simulink model "ActionPort_obs"  (Simulink 7.9)
settings: Solver=FixedStepDiscrete  SolverMode=SingleTasking  StartTime=0.0  StopTime=inf  RelTol=1e-3
PreLoadFcn:
  | if exist('tl_preloadfcn','file'), tl_preloadfcn(gcs,101); end
PostLoadFcn:
  | if exist('tl_postloadfcn','file'), tl_postloadfcn(gcs,101); end
InitFcn:
  | if exist('tlds_init','file'), tlds_init(gcs); end
StartFcn:
  | if exist('tlds_start','file'), tlds_start(gcs); end
StopFcn:
  | if exist('tlds_stop','file'), tlds_stop(gcs); end
(part 1 of 2)
PreSaveFcn:
  | if exist('tl_presavefcn','file'), tl_presavefcn(gcs); end
settings Model: TL_MAIN_DATA={'logopt',{'globalloggingmode',4},'date',736166.61526563659}  TLRevision=101  DS_PROJECTFILE=ActionPort_obs.dd  Creator=BTCJ_support  LastModifiedBy=developer  BufferReuse=off
settings OptimizationCC: BlockReduction=off  OptimizeBlockIOStorage=off  BufferReuse=off  ExpressionFolding=off  LocalBlockOutputs=off
settings DebuggingCC: StrictBusMsg=ErrorOnBusTreatedAsVector  NonBusSignalsTreatedAsBus=error
settings CodeAppCC: CustomSymbolStrType=$N$R$M_T
settings GRTTargetCC: CombineOutputUpdateFcns=off  GRTInterface=on

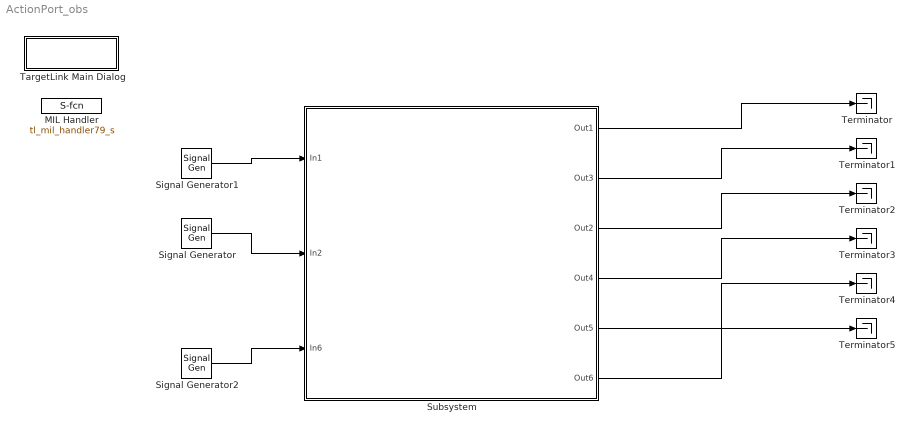
== system ActionPort_obs ==
  MIL Handler : S-Function  FunctionName=tl_mil_handler79_s  EnableBusSupport=off  mask(TL_MilHandler){data={'date',730486}}
      mask help: TargetLink MIL Handler
      mask init:
      | if get_param(0,'version') <= 8.2
      |     fname = sprintf('tl_mil_handler%d_s', 10*get_param(0,'Version'));
      | else
      | fname = sprintf('tl_mil_handler82_s');
      | end
      | set_param(gcbh,'FunctionName', fname, 'SFunctionModules','''''');
      settings: DeleteFcn=if exist('delete_tlblock','file')==2,delete_tlblock(gcbh);end  NameChangeFcn=if exist('rename_tlblock','file')==2,rename_tlblock(gcbh);end  OpenFcn=open_system(gcbh,'mask')
      mask Help: eval('if exist(''tl_online_help'',''file'') == 2, tl_online_help(''Topic'',get_param(gcbh,''MaskType'')),end')
      mask Display: disp('MIL Handler')
  Signal Generator : SignalGenerator
  Signal Generator1 : SignalGenerator
  Signal Generator2 : SignalGenerator
  Subsystem : Subsystem  Tag=TargetLink Simulation Frame
      settings: CopyFcn=if exist('tl_copyfcn','file'), tl_copyfcn(gcbh); end  NameChangeFcn=if exist('tl_framenamechangefcn','file'), tl_framenamechangefcn(gcbh); end
      settings: OpenFcn=|
      | if exist('open_tlsubsystem','file')
      |    open_tlsubsystem(gcbh);
      | else
      |    tlsubsystem = ...
      |       find_system(gcb, ...
      |       'LookUnderMasks','on', ...
      |       'FollowLinks','on', ...
      |       'Tag','MIL Subsystem');
      |    open_system(tlsubsystem);
      | end
      mask Type: TL_SimFrame
      mask Display: disp('TargetLink\nModel-\nin-the-loop\nmode')
  TargetLink Main Dialog : Subsystem  mask(TL_MainDialog){data=[]}
      mask help: TargetLink Main Dialog block: In full-featured mode it provides the main graphical user interface to TargetLink.
      mask init:
      | if exist('tl_get_blockset_mode','file')==2
      |    if strcmp(tl_get_blockset_mode,'full-featured')
      |       set_param(gcbh,'BackgroundColor','green');
      |    else
      |       set_param(gcbh,'BackgroundColor','[0.6,0.6,0.6]');
      |    end
      | else
      |    set_param(gcbh,'BackgroundColor','[0.6,0.6,0.6]');
      | end
      settings: CopyFcn=if exist('tl_copyfcn') == 2, tl_copyfcn(gcbh); end  OpenFcn=if exist('tl_open_blockdlg','file')==2,tl_open_blockdlg(gcbh);else,open_system(gcbh,'mask');end
      mask Help: eval('if exist(''tl_online_help'',''file'') == 2, tl_online_help(''Topic'',get_param(gcbh,''MaskType'')),end')
      mask Display: disp('TargetLink')
  Terminator{,1..5} (6 alike) : Terminator
  wires:
  Subsystem/1(Out1) -> Terminator/1
  Subsystem/2(Out3) -> Terminator1/1
  Subsystem/3(Out2) -> Terminator2/1
  Subsystem/4(Out4) -> Terminator3/1
  Subsystem/5(Out5) -> Terminator4/1
  Subsystem/6(Out6) -> Terminator5/1
  Signal Generator1/1 -> Subsystem/1(In1)
  Signal Generator/1 -> Subsystem/2(In2)
  Signal Generator2/1 -> Subsystem/3(In6)

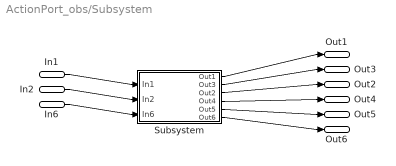
== system ActionPort_obs/Subsystem ==
  In1 : Inport
  In2 : Inport  Port=2
  In6 : Inport  Port=3
  Subsystem : Subsystem  Tag=struct('sfcnName','Subsystem_sf','subFunction','','srcSubsystem','')
      settings: OpenFcn=warndlg(get_param(gcb,'MaskHelp'),'Serious Warning');
      mask Type: TL_Enable
      mask Help: This subsystem keeps the TargetLink subsystem (subsystem with TargetLink blocks for production code generation), and is needed for the TargetLink simulation frame to work properly. DO NOT DELETE OR MODIFY IT!
  Out1 : Outport
  Out3 : Outport  Port=2
  Out2 : Outport  Port=3
  Out4 : Outport  Port=4
  Out5 : Outport  Port=5
  Out6 : Outport  Port=6
  wires:
  In1/1 -> Subsystem/1(In1)
  In2/1 -> Subsystem/2(In2)
  In6/1 -> Subsystem/3(In6)
  Subsystem/1(Out1) -> Out1/1
  Subsystem/2(Out3) -> Out3/1
  Subsystem/3(Out2) -> Out2/1
  Subsystem/4(Out4) -> Out4/1
  Subsystem/5(Out5) -> Out5/1
  Subsystem/6(Out6) -> Out6/1

== system ActionPort_obs/TargetLink Main Dialog ==
  dSPACE logo : Subsystem
      mask Display: image(ds_get_icon('dspace_logo_bg_white_l'))

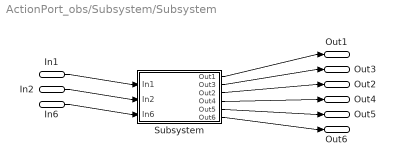
== system ActionPort_obs/Subsystem/Subsystem ==
  In1 : Inport
  In2 : Inport  Port=2
  In6 : Inport  Port=3
  Subsystem : Subsystem  Tag=MIL Subsystem  Description=a
      settings: CopyFcn=if exist('tl_copyfcn','file'), tl_copyfcn(gcbh); end  NameChangeFcn=if exist('tl_namechangefcn','file'), tl_namechangefcn(gcbh); end  DestroyFcn=if exist('update_tl_main_dlg','file'), update_tl_main_dlg('TL_subs_display'); end
      mask Type: MIL Subsystem
  Out1 : Outport
  Out3 : Outport  Port=2
  Out2 : Outport  Port=3
  Out4 : Outport  Port=4
  Out5 : Outport  Port=5
  Out6 : Outport  Port=6
  wires:
  In1/1 -> Subsystem/1(In1)
  In2/1 -> Subsystem/2(In2)
  In6/1 -> Subsystem/3(In6)
  Subsystem/1(Out1) -> Out1/1
  Subsystem/2(Out3) -> Out3/1
  Subsystem/3(Out2) -> Out2/1
  Subsystem/4(Out4) -> Out4/1
  Subsystem/5(Out5) -> Out5/1
  Subsystem/6(Out6) -> Out6/1

== system ActionPort_obs/TargetLink Main Dialog/dSPACE logo ==

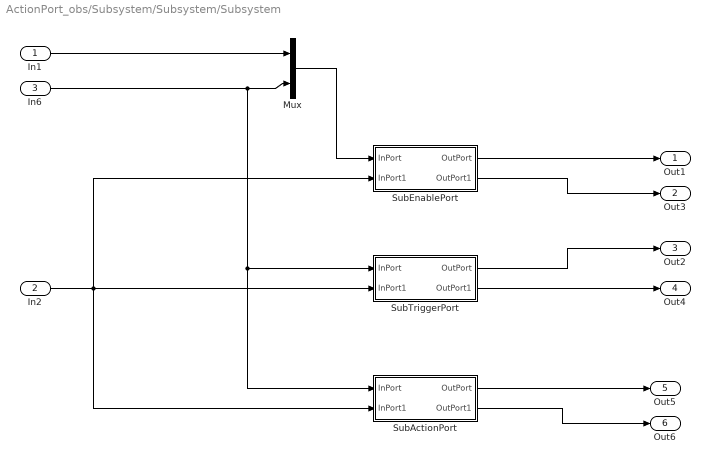
== system ActionPort_obs/Subsystem/Subsystem/Subsystem ==
  In1 : Inport  PortDimensions=1  mask(TL_Inport){data={'output',{'class','MBT_DISP'},'date',737456.38999608799}}
      settings: DeleteFcn=if exist('delete_tlblock','file')==2,delete_tlblock(gcbh);end  OpenFcn=if exist('tl_open_blockdlg','file')==2,tl_open_blockdlg(gcbh);else,open_system(gcbh,'parameter');end
      settings: CopyFcn=|
      | if exist('tl_reset_reviewflag','file')==2
      |     tl_reset_reviewflag(gcbh);
      | end
      | if exist('tl_check_ports','file')
      |     tl_check_ports(gcbh);
      | end
      settings: NameChangeFcn=|
      | if exist('rename_tlblock','file')==2,rename_tlblock(gcbh);end
      | if exist('tl_check_ports','file'), tl_check_ports(gcbh); end
      mask Help: eval(['if exist(''tl_online_help'',''file'') == 2, tl_online_help(''Topic'',''TL_Inport''),else, web([''jar:file:///'',matlabroot,''/help/toolbox/simulink/help.jar!/slref/' lower(get_param(gcbh,'Blocktype')) '.html''], ''-helpbrowser''),end'])
      mask Display: plot([0.2 0.35 NaN 0.65 0.8],[0 1 NaN 0 1]);
  In2 : Inport  Port=2  PortDimensions=1  mask(TL_Inport){data={'output',{'class','MBT_DISP'},'date',737456.38999631943}}
      settings: DeleteFcn=if exist('delete_tlblock','file')==2,delete_tlblock(gcbh);end  OpenFcn=if exist('tl_open_blockdlg','file')==2,tl_open_blockdlg(gcbh);else,open_system(gcbh,'parameter');end
      settings: CopyFcn=|
      | if exist('tl_reset_reviewflag','file')==2
      |     tl_reset_reviewflag(gcbh);
      | end
      | if exist('tl_check_ports','file')
      |     tl_check_ports(gcbh);
      | end
      settings: NameChangeFcn=|
      | if exist('rename_tlblock','file')==2,rename_tlblock(gcbh);end
      | if exist('tl_check_ports','file'), tl_check_ports(gcbh); end
      mask Help: eval(['if exist(''tl_online_help'',''file'') == 2, tl_online_help(''Topic'',''TL_Inport''),else, web([''jar:file:///'',matlabroot,''/help/toolbox/simulink/help.jar!/slref/' lower(get_param(gcbh,'Blocktype')) '.html''], ''-helpbrowser''),end'])
      mask Display: plot([0.2 0.35 NaN 0.65 0.8],[0 1 NaN 0 1]);
  In6 : Inport  Port=3  PortDimensions=1  mask(TL_Inport){data={'output',{'class','MBT_DISP'},'date',737456.38999655098}}
      settings: DeleteFcn=if exist('delete_tlblock','file')==2,delete_tlblock(gcbh);end  OpenFcn=if exist('tl_open_blockdlg','file')==2,tl_open_blockdlg(gcbh);else,open_system(gcbh,'parameter');end
      settings: CopyFcn=|
      | if exist('tl_reset_reviewflag','file')==2
      |     tl_reset_reviewflag(gcbh);
      | end
      | if exist('tl_check_ports','file')
      |     tl_check_ports(gcbh);
      | end
      settings: NameChangeFcn=|
      | if exist('rename_tlblock','file')==2,rename_tlblock(gcbh);end
      | if exist('tl_check_ports','file'), tl_check_ports(gcbh); end
      mask Help: eval(['if exist(''tl_online_help'',''file'') == 2, tl_online_help(''Topic'',''TL_Inport''),else, web([''jar:file:///'',matlabroot,''/help/toolbox/simulink/help.jar!/slref/' lower(get_param(gcbh,'Blocktype')) '.html''], ''-helpbrowser''),end'])
      mask Display: plot([0.2 0.35 NaN 0.65 0.8],[0 1 NaN 0 1]);
  Mux : Mux  Inputs=2
  SubActionPort : Subsystem
  SubEnablePort : Subsystem
  SubTriggerPort : Subsystem
  Out1 : Outport  mask(TL_Outport){data={'date',736495.67719833332}}
      settings: DeleteFcn=if exist('delete_tlblock','file')==2,delete_tlblock(gcbh);end  OpenFcn=if exist('tl_open_blockdlg','file')==2,tl_open_blockdlg(gcbh);else,open_system(gcbh,'parameter');end
      settings: CopyFcn=|
      | if exist('tl_reset_reviewflag','file')==2
      |     tl_reset_reviewflag(gcbh);
      | end
      | if exist('tl_check_ports','file')
      |     tl_check_ports(gcbh);
      | end
      settings: NameChangeFcn=|
      | if exist('rename_tlblock','file')==2,rename_tlblock(gcbh);end
      | if exist('tl_check_ports','file'), tl_check_ports(gcbh); end
      mask Help: eval(['if exist(''tl_online_help'',''file'') == 2, tl_online_help(''Topic'',''TL_Outport''),else, web([''jar:file:///'',matlabroot,''/help/toolbox/simulink/help.jar!/slref/' lower(get_param(gcbh,'Blocktype')) '.html''], ''-helpbrowser''),end'])
      mask Display: plot([0.2 0.35 NaN 0.65 0.8],[0 1 NaN 0 1]);
  Out3 : Outport  Port=2  mask(TL_Outport){data={'date',736495.6771985417}}
      settings: DeleteFcn=if exist('delete_tlblock','file')==2,delete_tlblock(gcbh);end  OpenFcn=if exist('tl_open_blockdlg','file')==2,tl_open_blockdlg(gcbh);else,open_system(gcbh,'parameter');end
      settings: CopyFcn=|
      | if exist('tl_reset_reviewflag','file')==2
      |     tl_reset_reviewflag(gcbh);
      | end
      | if exist('tl_check_ports','file')
      |     tl_check_ports(gcbh);
      | end
      settings: NameChangeFcn=|
      | if exist('rename_tlblock','file')==2,rename_tlblock(gcbh);end
      | if exist('tl_check_ports','file'), tl_check_ports(gcbh); end
      mask Help: eval(['if exist(''tl_online_help'',''file'') == 2, tl_online_help(''Topic'',''TL_Outport''),else, web([''jar:file:///'',matlabroot,''/help/toolbox/simulink/help.jar!/slref/' lower(get_param(gcbh,'Blocktype')) '.html''], ''-helpbrowser''),end'])
      mask Display: plot([0.2 0.35 NaN 0.65 0.8],[0 1 NaN 0 1]);
  Out2 : Outport  Port=3  mask(TL_Outport){data={'date',736495.67719871528}}
      settings: DeleteFcn=if exist('delete_tlblock','file')==2,delete_tlblock(gcbh);end  OpenFcn=if exist('tl_open_blockdlg','file')==2,tl_open_blockdlg(gcbh);else,open_system(gcbh,'parameter');end
      settings: CopyFcn=|
      | if exist('tl_reset_reviewflag','file')==2
      |     tl_reset_reviewflag(gcbh);
      | end
      | if exist('tl_check_ports','file')
      |     tl_check_ports(gcbh);
      | end
      settings: NameChangeFcn=|
      | if exist('rename_tlblock','file')==2,rename_tlblock(gcbh);end
      | if exist('tl_check_ports','file'), tl_check_ports(gcbh); end
      mask Help: eval(['if exist(''tl_online_help'',''file'') == 2, tl_online_help(''Topic'',''TL_Outport''),else, web([''jar:file:///'',matlabroot,''/help/toolbox/simulink/help.jar!/slref/' lower(get_param(gcbh,'Blocktype')) '.html''], ''-helpbrowser''),end'])
      mask Display: plot([0.2 0.35 NaN 0.65 0.8],[0 1 NaN 0 1]);
  Out4 : Outport  Port=4  mask(TL_Outport){data={'date',736495.67719890049}}
      settings: DeleteFcn=if exist('delete_tlblock','file')==2,delete_tlblock(gcbh);end  OpenFcn=if exist('tl_open_blockdlg','file')==2,tl_open_blockdlg(gcbh);else,open_system(gcbh,'parameter');end
      settings: CopyFcn=|
      | if exist('tl_reset_reviewflag','file')==2
      |     tl_reset_reviewflag(gcbh);
      | end
      | if exist('tl_check_ports','file')
      |     tl_check_ports(gcbh);
      | end
      settings: NameChangeFcn=|
      | if exist('rename_tlblock','file')==2,rename_tlblock(gcbh);end
      | if exist('tl_check_ports','file'), tl_check_ports(gcbh); end
      mask Help: eval(['if exist(''tl_online_help'',''file'') == 2, tl_online_help(''Topic'',''TL_Outport''),else, web([''jar:file:///'',matlabroot,''/help/toolbox/simulink/help.jar!/slref/' lower(get_param(gcbh,'Blocktype')) '.html''], ''-helpbrowser''),end'])
      mask Display: plot([0.2 0.35 NaN 0.65 0.8],[0 1 NaN 0 1]);
  Out5 : Outport  Port=5  mask(TL_Outport){data={'date',736495.67719907407}}
      settings: DeleteFcn=if exist('delete_tlblock','file')==2,delete_tlblock(gcbh);end  OpenFcn=if exist('tl_open_blockdlg','file')==2,tl_open_blockdlg(gcbh);else,open_system(gcbh,'parameter');end
      settings: CopyFcn=|
      | if exist('tl_reset_reviewflag','file')==2
      |     tl_reset_reviewflag(gcbh);
      | end
      | if exist('tl_check_ports','file')
      |     tl_check_ports(gcbh);
      | end
      settings: NameChangeFcn=|
      | if exist('rename_tlblock','file')==2,rename_tlblock(gcbh);end
      | if exist('tl_check_ports','file'), tl_check_ports(gcbh); end
      mask Help: eval(['if exist(''tl_online_help'',''file'') == 2, tl_online_help(''Topic'',''TL_Outport''),else, web([''jar:file:///'',matlabroot,''/help/toolbox/simulink/help.jar!/slref/' lower(get_param(gcbh,'Blocktype')) '.html''], ''-helpbrowser''),end'])
      mask Display: plot([0.2 0.35 NaN 0.65 0.8],[0 1 NaN 0 1]);
  Out6 : Outport  Port=6  mask(TL_Outport){data={'date',736495.67719924764}}
      settings: DeleteFcn=if exist('delete_tlblock','file')==2,delete_tlblock(gcbh);end  OpenFcn=if exist('tl_open_blockdlg','file')==2,tl_open_blockdlg(gcbh);else,open_system(gcbh,'parameter');end
      settings: CopyFcn=|
      | if exist('tl_reset_reviewflag','file')==2
      |     tl_reset_reviewflag(gcbh);
      | end
      | if exist('tl_check_ports','file')
      |     tl_check_ports(gcbh);
      | end
      settings: NameChangeFcn=|
      | if exist('rename_tlblock','file')==2,rename_tlblock(gcbh);end
      | if exist('tl_check_ports','file'), tl_check_ports(gcbh); end
      mask Help: eval(['if exist(''tl_online_help'',''file'') == 2, tl_online_help(''Topic'',''TL_Outport''),else, web([''jar:file:///'',matlabroot,''/help/toolbox/simulink/help.jar!/slref/' lower(get_param(gcbh,'Blocktype')) '.html''], ''-helpbrowser''),end'])
      mask Display: plot([0.2 0.35 NaN 0.65 0.8],[0 1 NaN 0 1]);
  wires:
  In6/1 -> SubActionPort/1(InPort), SubTriggerPort/1(InPort), Mux/2
  In1/1 -> Mux/1
  Mux/1 -> SubEnablePort/1(InPort)
  In2/1 -> SubActionPort/2(InPort1), SubTriggerPort/2(InPort1), SubEnablePort/2(InPort1)
  SubEnablePort/1(OutPort) -> Out1/1
  SubEnablePort/2(OutPort1) -> Out3/1
  SubTriggerPort/1(OutPort) -> Out2/1
  SubTriggerPort/2(OutPort1) -> Out4/1
  SubActionPort/1(OutPort) -> Out5/1
  SubActionPort/2(OutPort1) -> Out6/1

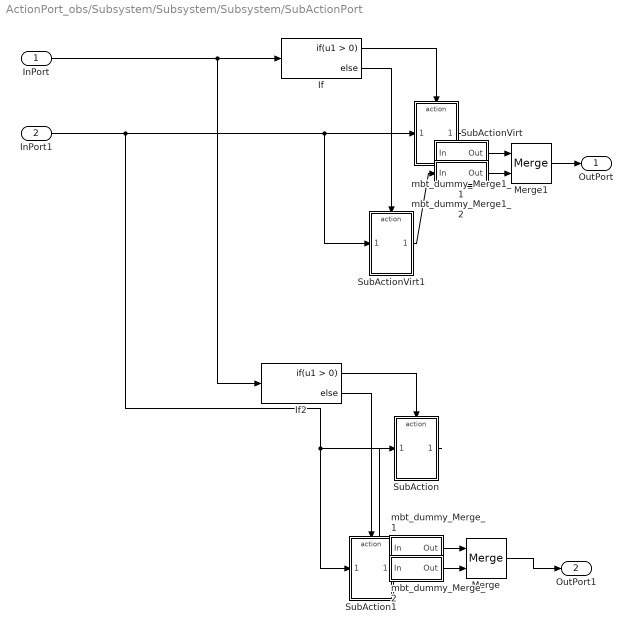
== system ActionPort_obs/Subsystem/Subsystem/Subsystem/SubActionPort ==
  InPort : Inport
      settings: CopyFcn=if exist('tl_reset_reviewflag') == 2, tl_reset_reviewflag(gcbh); end  DeleteFcn=if exist('delete_tlblock','file')==2,delete_tlblock(gcbh);end  NameChangeFcn=if exist('rename_tlblock','file')==2,rename_tlblock(gcbh);end  OpenFcn=if exist('tl_open_blockdlg','file')==2,tl_open_blockdlg(gcbh);else,open_system(gcbh,'parameter');end
  InPort1 : Inport  Port=2
      settings: CopyFcn=if exist('tl_reset_reviewflag') == 2, tl_reset_reviewflag(gcbh); end  DeleteFcn=if exist('delete_tlblock','file')==2,delete_tlblock(gcbh);end  NameChangeFcn=if exist('rename_tlblock','file')==2,rename_tlblock(gcbh);end  OpenFcn=if exist('tl_open_blockdlg','file')==2,tl_open_blockdlg(gcbh);else,open_system(gcbh,'parameter');end
  If : If
  If2 : If
  Merge : Merge  InitialOutput=[0]  mask(TL_Merge){data={'date',736495.67979597219}}
      settings: CopyFcn=if exist('tl_reset_reviewflag','file')==2,tl_reset_reviewflag(gcbh);end  DeleteFcn=if exist('delete_tlblock','file')==2,delete_tlblock(gcbh);end  NameChangeFcn=if exist('rename_tlblock','file')==2,rename_tlblock(gcbh);end  OpenFcn=if exist('tl_open_blockdlg','file')==2,tl_open_blockdlg(gcbh);else,open_system(gcbh,'parameter');end
      mask Help: eval(['if exist(''tl_online_help'',''file'') == 2, tl_online_help(''Topic'',''TL_Merge''),else, web([''jar:file:///'',matlabroot,''/help/toolbox/simulink/help.jar!/slref/' lower(get_param(gcbh,'Blocktype')) '.html''], ''-helpbrowser''),end'])
      mask Display: plot([-0.05, 1.05, NaN, -0.05, 1.05],[.01, .01, NaN, .99, .99])
  Merge1 : Merge  InitialOutput=[0]  mask(TL_Merge){data={'date',736495.679845787}}
      settings: CopyFcn=if exist('tl_reset_reviewflag','file')==2,tl_reset_reviewflag(gcbh);end  DeleteFcn=if exist('delete_tlblock','file')==2,delete_tlblock(gcbh);end  NameChangeFcn=if exist('rename_tlblock','file')==2,rename_tlblock(gcbh);end  OpenFcn=if exist('tl_open_blockdlg','file')==2,tl_open_blockdlg(gcbh);else,open_system(gcbh,'parameter');end
      mask Help: eval(['if exist(''tl_online_help'',''file'') == 2, tl_online_help(''Topic'',''TL_Merge''),else, web([''jar:file:///'',matlabroot,''/help/toolbox/simulink/help.jar!/slref/' lower(get_param(gcbh,'Blocktype')) '.html''], ''-helpbrowser''),end'])
      mask Display: plot([-0.05, 1.05, NaN, -0.05, 1.05],[.01, .01, NaN, .99, .99])
  SubAction : Subsystem
  SubAction1 : Subsystem
  SubActionVirt : Subsystem
  SubActionVirt1 : Subsystem
  mbt_dummy_Merge1_1 : Subsystem  Tag=et_enhanced_observability
      mask Type: MBT_DUMMY_BLOCK
      mask Display: text(0.1, 0.5, 'MBT_DUMMY')
  mbt_dummy_Merge1_2 : Subsystem  Tag=et_enhanced_observability
      mask Type: MBT_DUMMY_BLOCK
      mask Display: text(0.1, 0.5, 'MBT_DUMMY')
  mbt_dummy_Merge_1 : Subsystem  Tag=et_enhanced_observability
      mask Type: MBT_DUMMY_BLOCK
      mask Display: text(0.1, 0.5, 'MBT_DUMMY')
  mbt_dummy_Merge_2 : Subsystem  Tag=et_enhanced_observability
      mask Type: MBT_DUMMY_BLOCK
      mask Display: text(0.1, 0.5, 'MBT_DUMMY')
  OutPort : Outport
      settings: CopyFcn=if exist('tl_reset_reviewflag') == 2, tl_reset_reviewflag(gcbh); end  DeleteFcn=if exist('delete_tlblock','file')==2,delete_tlblock(gcbh);end  NameChangeFcn=if exist('rename_tlblock','file')==2,rename_tlblock(gcbh);end  OpenFcn=if exist('tl_open_blockdlg','file')==2,tl_open_blockdlg(gcbh);else,open_system(gcbh,'parameter');end
  OutPort1 : Outport  Port=2
      settings: CopyFcn=if exist('tl_reset_reviewflag') == 2, tl_reset_reviewflag(gcbh); end  DeleteFcn=if exist('delete_tlblock','file')==2,delete_tlblock(gcbh);end  NameChangeFcn=if exist('rename_tlblock','file')==2,rename_tlblock(gcbh);end  OpenFcn=if exist('tl_open_blockdlg','file')==2,tl_open_blockdlg(gcbh);else,open_system(gcbh,'parameter');end
  wires:
  InPort1/1 -> SubAction1/1(In1), SubAction/1(In1), SubActionVirt1/1(In1), SubActionVirt/1(In1)
  If2/1 -> SubAction/Action
  If/1 -> SubActionVirt/Action
  InPort/1 -> If2/1, If/1
  If2/2 -> SubAction1/Action
  Merge/1 -> OutPort1/1
  If/2 -> SubActionVirt1/Action
  Merge1/1 -> OutPort/1
  SubAction/1(Out1) -> mbt_dummy_Merge_1/1(In)
  mbt_dummy_Merge_1/1(Out) -> Merge/1
  SubAction1/1(Out1) -> mbt_dummy_Merge_2/1(In)
  mbt_dummy_Merge_2/1(Out) -> Merge/2
  SubActionVirt/1(Out1) -> mbt_dummy_Merge1_1/1(In)
  mbt_dummy_Merge1_1/1(Out) -> Merge1/1
  SubActionVirt1/1(Out1) -> mbt_dummy_Merge1_2/1(In)
  mbt_dummy_Merge1_2/1(Out) -> Merge1/2

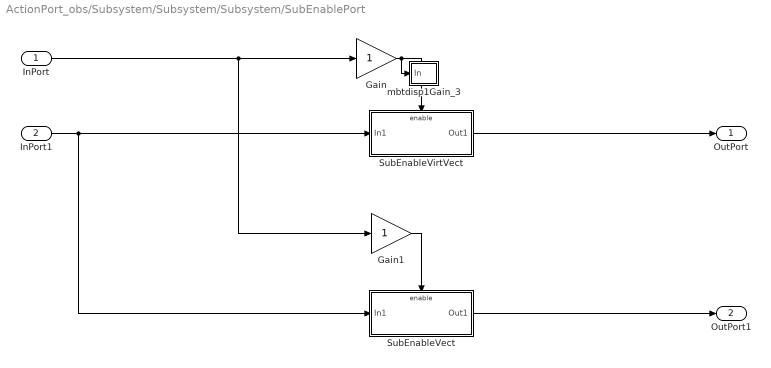
== system ActionPort_obs/Subsystem/Subsystem/Subsystem/SubEnablePort ==
  InPort : Inport
      settings: CopyFcn=if exist('tl_reset_reviewflag') == 2, tl_reset_reviewflag(gcbh); end  DeleteFcn=if exist('delete_tlblock','file')==2,delete_tlblock(gcbh);end  NameChangeFcn=if exist('rename_tlblock','file')==2,rename_tlblock(gcbh);end  OpenFcn=if exist('tl_open_blockdlg','file')==2,tl_open_blockdlg(gcbh);else,open_system(gcbh,'parameter');end
  InPort1 : Inport  Port=2
      settings: CopyFcn=if exist('tl_reset_reviewflag') == 2, tl_reset_reviewflag(gcbh); end  DeleteFcn=if exist('delete_tlblock','file')==2,delete_tlblock(gcbh);end  NameChangeFcn=if exist('rename_tlblock','file')==2,rename_tlblock(gcbh);end  OpenFcn=if exist('tl_open_blockdlg','file')==2,tl_open_blockdlg(gcbh);else,open_system(gcbh,'parameter');end
  Gain : Gain  mask(TL_Gain){data={'date',736495.67750707176}}
      settings: CopyFcn=if exist('tl_reset_reviewflag','file')==2,tl_reset_reviewflag(gcbh);end  DeleteFcn=if exist('delete_tlblock','file')==2,delete_tlblock(gcbh);end  NameChangeFcn=if exist('rename_tlblock','file')==2,rename_tlblock(gcbh);end  OpenFcn=if exist('tl_open_blockdlg','file')==2,tl_open_blockdlg(gcbh);else,open_system(gcbh,'parameter');end
      mask Help: eval(['if exist(''tl_online_help'',''file'') == 2, tl_online_help(''Topic'',''TL_Gain''),else, web([''jar:file:///'',matlabroot,''/help/toolbox/simulink/help.jar!/slref/' lower(get_param(gcbh,'Blocktype')) '.html''], ''-helpbrowser''),end'])
      mask Display: plot([0, .9, 0],[.05, .5, .95])
  Gain1 : Gain  mask(TL_Gain){data={'date',736495.67750723381}}
      settings: CopyFcn=if exist('tl_reset_reviewflag','file')==2,tl_reset_reviewflag(gcbh);end  DeleteFcn=if exist('delete_tlblock','file')==2,delete_tlblock(gcbh);end  NameChangeFcn=if exist('rename_tlblock','file')==2,rename_tlblock(gcbh);end  OpenFcn=if exist('tl_open_blockdlg','file')==2,tl_open_blockdlg(gcbh);else,open_system(gcbh,'parameter');end
      mask Help: eval(['if exist(''tl_online_help'',''file'') == 2, tl_online_help(''Topic'',''TL_Gain''),else, web([''jar:file:///'',matlabroot,''/help/toolbox/simulink/help.jar!/slref/' lower(get_param(gcbh,'Blocktype')) '.html''], ''-helpbrowser''),end'])
      mask Display: plot([0, .9, 0],[.05, .5, .95])
  SubEnableVect : Subsystem
  SubEnableVirtVect : Subsystem
  mbtdisp1Gain_3 : Subsystem  Tag=et_enhanced_observability
      mask Type: MBT_DISP_BLOCK
      mask Display: text(0.1, 0.5, 'MBT_DISP')
  OutPort : Outport
      settings: CopyFcn=if exist('tl_reset_reviewflag') == 2, tl_reset_reviewflag(gcbh); end  DeleteFcn=if exist('delete_tlblock','file')==2,delete_tlblock(gcbh);end  NameChangeFcn=if exist('rename_tlblock','file')==2,rename_tlblock(gcbh);end  OpenFcn=if exist('tl_open_blockdlg','file')==2,tl_open_blockdlg(gcbh);else,open_system(gcbh,'parameter');end
  OutPort1 : Outport  Port=2
      settings: CopyFcn=if exist('tl_reset_reviewflag') == 2, tl_reset_reviewflag(gcbh); end  DeleteFcn=if exist('delete_tlblock','file')==2,delete_tlblock(gcbh);end  NameChangeFcn=if exist('rename_tlblock','file')==2,rename_tlblock(gcbh);end  OpenFcn=if exist('tl_open_blockdlg','file')==2,tl_open_blockdlg(gcbh);else,open_system(gcbh,'parameter');end
  wires:
  InPort1/1 -> SubEnableVect/1(In1), SubEnableVirtVect/1(In1)
  InPort/1 -> Gain1/1, Gain/1
  SubEnableVirtVect/1(Out1) -> OutPort/1
  SubEnableVect/1(Out1) -> OutPort1/1
  Gain/1 -> SubEnableVirtVect/Enable, mbtdisp1Gain_3/1(In)
  Gain1/1 -> SubEnableVect/Enable

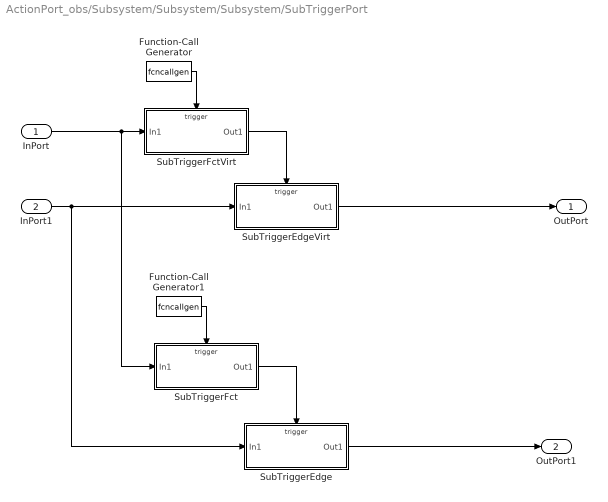
== system ActionPort_obs/Subsystem/Subsystem/Subsystem/SubTriggerPort ==
  InPort : Inport
      settings: CopyFcn=if exist('tl_reset_reviewflag') == 2, tl_reset_reviewflag(gcbh); end  DeleteFcn=if exist('delete_tlblock','file')==2,delete_tlblock(gcbh);end  NameChangeFcn=if exist('rename_tlblock','file')==2,rename_tlblock(gcbh);end  OpenFcn=if exist('tl_open_blockdlg','file')==2,tl_open_blockdlg(gcbh);else,open_system(gcbh,'parameter');end
  InPort1 : Inport  Port=2
      settings: CopyFcn=if exist('tl_reset_reviewflag') == 2, tl_reset_reviewflag(gcbh); end  DeleteFcn=if exist('delete_tlblock','file')==2,delete_tlblock(gcbh);end  NameChangeFcn=if exist('rename_tlblock','file')==2,rename_tlblock(gcbh);end  OpenFcn=if exist('tl_open_blockdlg','file')==2,tl_open_blockdlg(gcbh);else,open_system(gcbh,'parameter');end
  Function-Call Generator : S-Function  FunctionName=fcncallgen  Parameters=sample_time,numberOfIterations  EnableBusSupport=off  mask(Function-Call Generator){sample_time=2, numberOfIterations=1}
      mask prompts: sample_time "Simulink:masks:SampleTime_MP"; numberOfIterations "Simulink:masks:NumberOfIterations_MP"
      mask help: Simulink:masks:FunctionCallGenerator_MD
      mask init:
      | if ~isempty(numberOfIterations) & length(numberOfIterations) == 1 & (numberOfIterations > 1),
      | str=sprintf('iterate I = 1:%d',numberOfIterations);
      | else, str = 'f()';
      | end;
      mask Help: This block executes a function-call subsystem at the rate specified by the sample time and a specified number of times.
      mask Display: disp(str)
  Function-Call Generator1 : S-Function  FunctionName=fcncallgen  Parameters=sample_time,numberOfIterations  EnableBusSupport=off  mask(Function-Call Generator){sample_time=2, numberOfIterations=1}
      mask prompts: sample_time "Simulink:masks:SampleTime_MP"; numberOfIterations "Simulink:masks:NumberOfIterations_MP"
      mask help: Simulink:masks:FunctionCallGenerator_MD
      mask init:
      | if ~isempty(numberOfIterations) & length(numberOfIterations) == 1 & (numberOfIterations > 1),
      | str=sprintf('iterate I = 1:%d',numberOfIterations);
      | else, str = 'f()';
      | end;
      mask Help: This block executes a function-call subsystem at the rate specified by the sample time and a specified number of times.
      mask Display: disp(str)
  SubTriggerEdge : Subsystem
  SubTriggerEdgeVirt : Subsystem
  SubTriggerFct : Subsystem
  SubTriggerFctVirt : Subsystem
  OutPort : Outport
      settings: CopyFcn=if exist('tl_reset_reviewflag') == 2, tl_reset_reviewflag(gcbh); end  DeleteFcn=if exist('delete_tlblock','file')==2,delete_tlblock(gcbh);end  NameChangeFcn=if exist('rename_tlblock','file')==2,rename_tlblock(gcbh);end  OpenFcn=if exist('tl_open_blockdlg','file')==2,tl_open_blockdlg(gcbh);else,open_system(gcbh,'parameter');end
  OutPort1 : Outport  Port=2
      settings: CopyFcn=if exist('tl_reset_reviewflag') == 2, tl_reset_reviewflag(gcbh); end  DeleteFcn=if exist('delete_tlblock','file')==2,delete_tlblock(gcbh);end  NameChangeFcn=if exist('rename_tlblock','file')==2,rename_tlblock(gcbh);end  OpenFcn=if exist('tl_open_blockdlg','file')==2,tl_open_blockdlg(gcbh);else,open_system(gcbh,'parameter');end
  wires:
  InPort/1 -> SubTriggerFct/1(In1), SubTriggerFctVirt/1(In1)
  SubTriggerFctVirt/1(Out1) -> SubTriggerEdgeVirt/Trigger
  Function-Call Generator/1 -> SubTriggerFctVirt/Trigger
  SubTriggerEdgeVirt/1(Out1) -> OutPort/1
  SubTriggerFct/1(Out1) -> SubTriggerEdge/Trigger
  Function-Call Generator1/1 -> SubTriggerFct/Trigger
  SubTriggerEdge/1(Out1) -> OutPort1/1
  InPort1/1 -> SubTriggerEdge/1(In1), SubTriggerEdgeVirt/1(In1)

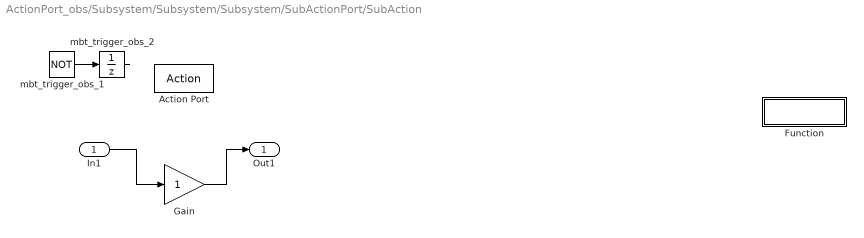
== system ActionPort_obs/Subsystem/Subsystem/Subsystem/SubActionPort/SubAction ==
  In1 : Inport
  Action Port : ActionPort  ActionType=then
  Function : Subsystem  LoadFcn=if exist('tl_loadfcn','file')==2,tl_loadfcn(gcbh);end  mask(TL_Function){data={'date',730486}}
      mask help: TargetLink Function block: It is used to generate code for a subsystem in a separate C function. In full-featured mode it provides an graphical user interface.
      mask init:
      | hBlock = gcbh;
      | if exist('tl_get_blockset_mode','file')==2
      |    if strcmp(tl_get_blockset_mode,'full-featured')
      |       set_param(hBlock,'BackgroundColor','green');
      |    else
      |       set_param(hBlock,'BackgroundColor','[0.6,0.6,0.6]');
      |    end
      | else
      |    set_param(hBlock,'BackgroundColor','[0.6,0.6,0.6]');
      | end
      |  
      | if exist('tl_add_swcparameter','file')==2
      |     tl_add_swcparameter(hBlock);
      | end
      settings: DeleteFcn=if exist('delete_tlblock','file')==2,delete_tlblock(gcbh);end  NameChangeFcn=if exist('rename_tlblock','file')==2,rename_tlblock(gcbh);end  OpenFcn=if exist('tl_open_blockdlg','file')==2,tl_open_blockdlg(gcbh);else,open_system(gcbh,'mask');end
      mask Help: eval('if exist(''tl_online_help'',''file'') == 2, tl_online_help(''Topic'',get_param(gcbh,''MaskType'')),end')
      mask Display: disp('FUNCTION')
  Gain : Gain  mask(TL_Gain){data={'date',736495.67856915505}}
      settings: CopyFcn=if exist('tl_reset_reviewflag','file')==2,tl_reset_reviewflag(gcbh);end  DeleteFcn=if exist('delete_tlblock','file')==2,delete_tlblock(gcbh);end  NameChangeFcn=if exist('rename_tlblock','file')==2,rename_tlblock(gcbh);end  OpenFcn=if exist('tl_open_blockdlg','file')==2,tl_open_blockdlg(gcbh);else,open_system(gcbh,'parameter');end
      mask Help: eval(['if exist(''tl_online_help'',''file'') == 2, tl_online_help(''Topic'',''TL_Gain''),else, web([''jar:file:///'',matlabroot,''/help/toolbox/simulink/help.jar!/slref/' lower(get_param(gcbh,'Blocktype')) '.html''], ''-helpbrowser''),end'])
      mask Display: plot([0, .9, 0],[.05, .5, .95])
  mbt_trigger_obs_1 : Logic  Tag=mbt_add_trigger_obs  Operator=NOT  Inputs=1  AllPortsSameDT=off  OutDataTypeStr=boolean  mask(TL_LogicalOperator){data={'output',{'class','MBT_DISP'},'date',737456.38998781249}}
      settings: DeleteFcn=if exist('delete_tlblock','file')==2,delete_tlblock(gcbh);end  NameChangeFcn=if exist('rename_tlblock','file')==2,rename_tlblock(gcbh);end  OpenFcn=if exist('tl_open_blockdlg','file')==2,tl_open_blockdlg(gcbh);else,open_system(gcbh,'parameter');end
      mask Help: eval(['if exist(''tl_online_help'',''file'') == 2, tl_online_help(''Topic'',''TL_LogicalOperator''),else, web([''jar:file:///'',matlabroot,''/help/toolbox/simulink/help.jar!/slref/' lower(get_param(gcbh,'Blocktype')) '.html''], ''-helpbrowser''),end'])
      mask Display: plot([-0.05, 1.05, NaN, -0.05, 1.05],[.01, .01, NaN, .99, .99])
  mbt_trigger_obs_2 : UnitDelay  Tag=mbt_add_trigger_obs  SampleTime=-1  mask(TL_UnitDelay){data={'output',{'type','Bool'},'state',{'type','Bool'},'date',737456.38998839119}}
      settings: CopyFcn=if exist('tl_reset_reviewflag') == 2, tl_reset_reviewflag(gcbh); end  DeleteFcn=if exist('delete_tlblock','file')==2,delete_tlblock(gcbh);end  NameChangeFcn=if exist('rename_tlblock','file')==2,rename_tlblock(gcbh);end  OpenFcn=if exist('tl_open_blockdlg','file')==2,tl_open_blockdlg(gcbh);else,open_system(gcbh,'parameter');end
      mask Help: eval(['if exist(''tl_online_help'',''file'') == 2, tl_online_help(''Topic'',''TL_UnitDelay''),else, web([''jar:file:///'',matlabroot,''/help/toolbox/simulink/help.jar!/slref/' lower(get_param(gcbh,'Blocktype')) '.html''], ''-helpbrowser''),end'])
      mask Display: plot([-0.05, 1.05, NaN, -0.05, 1.05],[.01, .01, NaN, .99, .99])
  Out1 : Outport  InitialOutput=0
  wires:
  In1/1 -> Gain/1
  Gain/1 -> Out1/1
  mbt_trigger_obs_1/1 -> mbt_trigger_obs_2/1
  mbt_trigger_obs_2/1 -> mbt_trigger_obs_1/1

== system ActionPort_obs/Subsystem/Subsystem/Subsystem/SubActionPort/SubAction1 ==
  In1 : Inport
  Action Port : ActionPort  ActionType=else
  Function : Subsystem  LoadFcn=if exist('tl_loadfcn','file')==2,tl_loadfcn(gcbh);end  mask(TL_Function){data={'date',730486}}
      mask help: TargetLink Function block: It is used to generate code for a subsystem in a separate C function. In full-featured mode it provides an graphical user interface.
      mask init: same as ActionPort_obs/Subsystem/Subsystem/Subsystem/SubActionPort/SubAction/Function
      settings: DeleteFcn=if exist('delete_tlblock','file')==2,delete_tlblock(gcbh);end  NameChangeFcn=if exist('rename_tlblock','file')==2,rename_tlblock(gcbh);end  OpenFcn=if exist('tl_open_blockdlg','file')==2,tl_open_blockdlg(gcbh);else,open_system(gcbh,'mask');end
      mask Help: eval('if exist(''tl_online_help'',''file'') == 2, tl_online_help(''Topic'',get_param(gcbh,''MaskType'')),end')
      mask Display: disp('FUNCTION')
  Gain : Gain  mask(TL_Gain){data={'date',736495.678753588}}
      settings: CopyFcn=if exist('tl_reset_reviewflag','file')==2,tl_reset_reviewflag(gcbh);end  DeleteFcn=if exist('delete_tlblock','file')==2,delete_tlblock(gcbh);end  NameChangeFcn=if exist('rename_tlblock','file')==2,rename_tlblock(gcbh);end  OpenFcn=if exist('tl_open_blockdlg','file')==2,tl_open_blockdlg(gcbh);else,open_system(gcbh,'parameter');end
      mask Help: eval(['if exist(''tl_online_help'',''file'') == 2, tl_online_help(''Topic'',''TL_Gain''),else, web([''jar:file:///'',matlabroot,''/help/toolbox/simulink/help.jar!/slref/' lower(get_param(gcbh,'Blocktype')) '.html''], ''-helpbrowser''),end'])
      mask Display: plot([0, .9, 0],[.05, .5, .95])
  mbt_trigger_obs_1 : Logic  Tag=mbt_add_trigger_obs  Operator=NOT  Inputs=1  AllPortsSameDT=off  OutDataTypeStr=boolean  mask(TL_LogicalOperator){data={'output',{'class','MBT_DISP'},'date',737456.38999358797}}
      settings: DeleteFcn=if exist('delete_tlblock','file')==2,delete_tlblock(gcbh);end  NameChangeFcn=if exist('rename_tlblock','file')==2,rename_tlblock(gcbh);end  OpenFcn=if exist('tl_open_blockdlg','file')==2,tl_open_blockdlg(gcbh);else,open_system(gcbh,'parameter');end
      mask Help: eval(['if exist(''tl_online_help'',''file'') == 2, tl_online_help(''Topic'',''TL_LogicalOperator''),else, web([''jar:file:///'',matlabroot,''/help/toolbox/simulink/help.jar!/slref/' lower(get_param(gcbh,'Blocktype')) '.html''], ''-helpbrowser''),end'])
      mask Display: plot([-0.05, 1.05, NaN, -0.05, 1.05],[.01, .01, NaN, .99, .99])
  mbt_trigger_obs_2 : UnitDelay  Tag=mbt_add_trigger_obs  SampleTime=-1  mask(TL_UnitDelay){data={'output',{'type','Bool'},'state',{'type','Bool'},'date',737456.38999415515}}
      settings: CopyFcn=if exist('tl_reset_reviewflag') == 2, tl_reset_reviewflag(gcbh); end  DeleteFcn=if exist('delete_tlblock','file')==2,delete_tlblock(gcbh);end  NameChangeFcn=if exist('rename_tlblock','file')==2,rename_tlblock(gcbh);end  OpenFcn=if exist('tl_open_blockdlg','file')==2,tl_open_blockdlg(gcbh);else,open_system(gcbh,'parameter');end
      mask Help: eval(['if exist(''tl_online_help'',''file'') == 2, tl_online_help(''Topic'',''TL_UnitDelay''),else, web([''jar:file:///'',matlabroot,''/help/toolbox/simulink/help.jar!/slref/' lower(get_param(gcbh,'Blocktype')) '.html''], ''-helpbrowser''),end'])
      mask Display: plot([-0.05, 1.05, NaN, -0.05, 1.05],[.01, .01, NaN, .99, .99])
  Out1 : Outport  InitialOutput=0
  wires:
  In1/1 -> Gain/1
  Gain/1 -> Out1/1
  mbt_trigger_obs_1/1 -> mbt_trigger_obs_2/1
  mbt_trigger_obs_2/1 -> mbt_trigger_obs_1/1

== system ActionPort_obs/Subsystem/Subsystem/Subsystem/SubActionPort/SubActionVirt ==
  In1 : Inport
  Action Port : ActionPort  ActionType=then
  Gain : Gain  mask(TL_Gain){data={'date',736495.67814083328}}
      settings: CopyFcn=if exist('tl_reset_reviewflag','file')==2,tl_reset_reviewflag(gcbh);end  DeleteFcn=if exist('delete_tlblock','file')==2,delete_tlblock(gcbh);end  NameChangeFcn=if exist('rename_tlblock','file')==2,rename_tlblock(gcbh);end  OpenFcn=if exist('tl_open_blockdlg','file')==2,tl_open_blockdlg(gcbh);else,open_system(gcbh,'parameter');end
      mask Help: eval(['if exist(''tl_online_help'',''file'') == 2, tl_online_help(''Topic'',''TL_Gain''),else, web([''jar:file:///'',matlabroot,''/help/toolbox/simulink/help.jar!/slref/' lower(get_param(gcbh,'Blocktype')) '.html''], ''-helpbrowser''),end'])
      mask Display: plot([0, .9, 0],[.05, .5, .95])
  mbt_trigger_obs_1 : Logic  Tag=mbt_add_trigger_obs  Operator=NOT  Inputs=1  AllPortsSameDT=off  OutDataTypeStr=boolean  mask(TL_LogicalOperator){data={'output',{'class','MBT_DISP'},'date',737456.38998442132}}
      settings: DeleteFcn=if exist('delete_tlblock','file')==2,delete_tlblock(gcbh);end  NameChangeFcn=if exist('rename_tlblock','file')==2,rename_tlblock(gcbh);end  OpenFcn=if exist('tl_open_blockdlg','file')==2,tl_open_blockdlg(gcbh);else,open_system(gcbh,'parameter');end
      mask Help: eval(['if exist(''tl_online_help'',''file'') == 2, tl_online_help(''Topic'',''TL_LogicalOperator''),else, web([''jar:file:///'',matlabroot,''/help/toolbox/simulink/help.jar!/slref/' lower(get_param(gcbh,'Blocktype')) '.html''], ''-helpbrowser''),end'])
      mask Display: plot([-0.05, 1.05, NaN, -0.05, 1.05],[.01, .01, NaN, .99, .99])
  mbt_trigger_obs_2 : UnitDelay  Tag=mbt_add_trigger_obs  SampleTime=-1  mask(TL_UnitDelay){data={'output',{'type','Bool'},'state',{'type','Bool'},'date',737456.38998500002}}
      settings: CopyFcn=if exist('tl_reset_reviewflag') == 2, tl_reset_reviewflag(gcbh); end  DeleteFcn=if exist('delete_tlblock','file')==2,delete_tlblock(gcbh);end  NameChangeFcn=if exist('rename_tlblock','file')==2,rename_tlblock(gcbh);end  OpenFcn=if exist('tl_open_blockdlg','file')==2,tl_open_blockdlg(gcbh);else,open_system(gcbh,'parameter');end
      mask Help: eval(['if exist(''tl_online_help'',''file'') == 2, tl_online_help(''Topic'',''TL_UnitDelay''),else, web([''jar:file:///'',matlabroot,''/help/toolbox/simulink/help.jar!/slref/' lower(get_param(gcbh,'Blocktype')) '.html''], ''-helpbrowser''),end'])
      mask Display: plot([-0.05, 1.05, NaN, -0.05, 1.05],[.01, .01, NaN, .99, .99])
  Out1 : Outport  InitialOutput=0
  wires:
  In1/1 -> Gain/1
  Gain/1 -> Out1/1
  mbt_trigger_obs_1/1 -> mbt_trigger_obs_2/1
  mbt_trigger_obs_2/1 -> mbt_trigger_obs_1/1

== system ActionPort_obs/Subsystem/Subsystem/Subsystem/SubActionPort/SubActionVirt1 ==
  In1 : Inport
  Action Port : ActionPort  ActionType=else
  Gain : Gain  mask(TL_Gain){data={'date',736495.67832232639}}
      settings: CopyFcn=if exist('tl_reset_reviewflag','file')==2,tl_reset_reviewflag(gcbh);end  DeleteFcn=if exist('delete_tlblock','file')==2,delete_tlblock(gcbh);end  NameChangeFcn=if exist('rename_tlblock','file')==2,rename_tlblock(gcbh);end  OpenFcn=if exist('tl_open_blockdlg','file')==2,tl_open_blockdlg(gcbh);else,open_system(gcbh,'parameter');end
      mask Help: eval(['if exist(''tl_online_help'',''file'') == 2, tl_online_help(''Topic'',''TL_Gain''),else, web([''jar:file:///'',matlabroot,''/help/toolbox/simulink/help.jar!/slref/' lower(get_param(gcbh,'Blocktype')) '.html''], ''-helpbrowser''),end'])
      mask Display: plot([0, .9, 0],[.05, .5, .95])
  mbt_trigger_obs_1 : Logic  Tag=mbt_add_trigger_obs  Operator=NOT  Inputs=1  AllPortsSameDT=off  OutDataTypeStr=boolean  mask(TL_LogicalOperator){data={'output',{'class','MBT_DISP'},'date',737456.38999011577}}
      settings: DeleteFcn=if exist('delete_tlblock','file')==2,delete_tlblock(gcbh);end  NameChangeFcn=if exist('rename_tlblock','file')==2,rename_tlblock(gcbh);end  OpenFcn=if exist('tl_open_blockdlg','file')==2,tl_open_blockdlg(gcbh);else,open_system(gcbh,'parameter');end
      mask Help: eval(['if exist(''tl_online_help'',''file'') == 2, tl_online_help(''Topic'',''TL_LogicalOperator''),else, web([''jar:file:///'',matlabroot,''/help/toolbox/simulink/help.jar!/slref/' lower(get_param(gcbh,'Blocktype')) '.html''], ''-helpbrowser''),end'])
      mask Display: plot([-0.05, 1.05, NaN, -0.05, 1.05],[.01, .01, NaN, .99, .99])
  mbt_trigger_obs_2 : UnitDelay  Tag=mbt_add_trigger_obs  SampleTime=-1  mask(TL_UnitDelay){data={'output',{'type','Bool'},'state',{'type','Bool'},'date',737456.38999069447}}
      settings: CopyFcn=if exist('tl_reset_reviewflag') == 2, tl_reset_reviewflag(gcbh); end  DeleteFcn=if exist('delete_tlblock','file')==2,delete_tlblock(gcbh);end  NameChangeFcn=if exist('rename_tlblock','file')==2,rename_tlblock(gcbh);end  OpenFcn=if exist('tl_open_blockdlg','file')==2,tl_open_blockdlg(gcbh);else,open_system(gcbh,'parameter');end
      mask Help: eval(['if exist(''tl_online_help'',''file'') == 2, tl_online_help(''Topic'',''TL_UnitDelay''),else, web([''jar:file:///'',matlabroot,''/help/toolbox/simulink/help.jar!/slref/' lower(get_param(gcbh,'Blocktype')) '.html''], ''-helpbrowser''),end'])
      mask Display: plot([-0.05, 1.05, NaN, -0.05, 1.05],[.01, .01, NaN, .99, .99])
  Out1 : Outport  InitialOutput=0
  wires:
  In1/1 -> Gain/1
  Gain/1 -> Out1/1
  mbt_trigger_obs_1/1 -> mbt_trigger_obs_2/1
  mbt_trigger_obs_2/1 -> mbt_trigger_obs_1/1

== system ActionPort_obs/Subsystem/Subsystem/Subsystem/SubActionPort/mbt_dummy_Merge1_1 ==
  In : Inport  Tag=et_enhanced_observability
  Data Type Conversion : DataTypeConversion  Tag=et_enhanced_observability
  Out : Outport  Tag=et_enhanced_observability
  wires:
  In/1 -> Data Type Conversion/1
  Data Type Conversion/1 -> Out/1

== system ActionPort_obs/Subsystem/Subsystem/Subsystem/SubActionPort/mbt_dummy_Merge1_2 ==
  In : Inport  Tag=et_enhanced_observability
  Data Type Conversion : DataTypeConversion  Tag=et_enhanced_observability
  Out : Outport  Tag=et_enhanced_observability
  wires:
  In/1 -> Data Type Conversion/1
  Data Type Conversion/1 -> Out/1

== system ActionPort_obs/Subsystem/Subsystem/Subsystem/SubActionPort/mbt_dummy_Merge_1 ==
  In : Inport  Tag=et_enhanced_observability
  Data Type Conversion : DataTypeConversion  Tag=et_enhanced_observability
  Out : Outport  Tag=et_enhanced_observability
  wires:
  In/1 -> Data Type Conversion/1
  Data Type Conversion/1 -> Out/1

== system ActionPort_obs/Subsystem/Subsystem/Subsystem/SubActionPort/mbt_dummy_Merge_2 ==
  In : Inport  Tag=et_enhanced_observability
  Data Type Conversion : DataTypeConversion  Tag=et_enhanced_observability
  Out : Outport  Tag=et_enhanced_observability
  wires:
  In/1 -> Data Type Conversion/1
  Data Type Conversion/1 -> Out/1

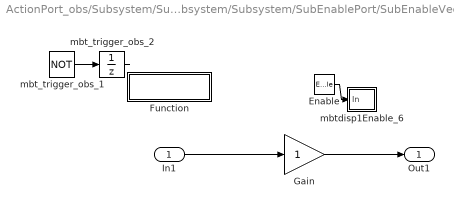
== system ActionPort_obs/Subsystem/Subsystem/Subsystem/SubEnablePort/SubEnableVect ==
  In1 : Inport
  Enable : EnablePort  ShowOutputPort=on
  Function : Subsystem  LoadFcn=if exist('tl_loadfcn','file')==2,tl_loadfcn(gcbh);end  mask(TL_Function){data={'date',730486}}
      mask help: TargetLink Function block: It is used to generate code for a subsystem in a separate C function. In full-featured mode it provides an graphical user interface.
      mask init: same as ActionPort_obs/Subsystem/Subsystem/Subsystem/SubActionPort/SubAction/Function
      settings: DeleteFcn=if exist('delete_tlblock','file')==2,delete_tlblock(gcbh);end  NameChangeFcn=if exist('rename_tlblock','file')==2,rename_tlblock(gcbh);end  OpenFcn=if exist('tl_open_blockdlg','file')==2,tl_open_blockdlg(gcbh);else,open_system(gcbh,'mask');end
      mask Help: eval('if exist(''tl_online_help'',''file'') == 2, tl_online_help(''Topic'',get_param(gcbh,''MaskType'')),end')
      mask Display: disp('FUNCTION')
  Gain : Gain  mask(TL_Gain){data={'date',736495.67765583331}}
      settings: CopyFcn=if exist('tl_reset_reviewflag','file')==2,tl_reset_reviewflag(gcbh);end  DeleteFcn=if exist('delete_tlblock','file')==2,delete_tlblock(gcbh);end  NameChangeFcn=if exist('rename_tlblock','file')==2,rename_tlblock(gcbh);end  OpenFcn=if exist('tl_open_blockdlg','file')==2,tl_open_blockdlg(gcbh);else,open_system(gcbh,'parameter');end
      mask Help: eval(['if exist(''tl_online_help'',''file'') == 2, tl_online_help(''Topic'',''TL_Gain''),else, web([''jar:file:///'',matlabroot,''/help/toolbox/simulink/help.jar!/slref/' lower(get_param(gcbh,'Blocktype')) '.html''], ''-helpbrowser''),end'])
      mask Display: plot([0, .9, 0],[.05, .5, .95])
  mbt_trigger_obs_1 : Logic  Tag=mbt_add_trigger_obs  Operator=NOT  Inputs=1  AllPortsSameDT=off  OutDataTypeStr=boolean  mask(TL_LogicalOperator){data={'output',{'class','MBT_DISP'},'date',737456.38998556708}}
      settings: DeleteFcn=if exist('delete_tlblock','file')==2,delete_tlblock(gcbh);end  NameChangeFcn=if exist('rename_tlblock','file')==2,rename_tlblock(gcbh);end  OpenFcn=if exist('tl_open_blockdlg','file')==2,tl_open_blockdlg(gcbh);else,open_system(gcbh,'parameter');end
      mask Help: eval(['if exist(''tl_online_help'',''file'') == 2, tl_online_help(''Topic'',''TL_LogicalOperator''),else, web([''jar:file:///'',matlabroot,''/help/toolbox/simulink/help.jar!/slref/' lower(get_param(gcbh,'Blocktype')) '.html''], ''-helpbrowser''),end'])
      mask Display: plot([-0.05, 1.05, NaN, -0.05, 1.05],[.01, .01, NaN, .99, .99])
  mbt_trigger_obs_2 : UnitDelay  Tag=mbt_add_trigger_obs  SampleTime=-1  mask(TL_UnitDelay){data={'output',{'type','Bool'},'state',{'type','Bool'},'date',737456.38998611108}}
      settings: CopyFcn=if exist('tl_reset_reviewflag') == 2, tl_reset_reviewflag(gcbh); end  DeleteFcn=if exist('delete_tlblock','file')==2,delete_tlblock(gcbh);end  NameChangeFcn=if exist('rename_tlblock','file')==2,rename_tlblock(gcbh);end  OpenFcn=if exist('tl_open_blockdlg','file')==2,tl_open_blockdlg(gcbh);else,open_system(gcbh,'parameter');end
      mask Help: eval(['if exist(''tl_online_help'',''file'') == 2, tl_online_help(''Topic'',''TL_UnitDelay''),else, web([''jar:file:///'',matlabroot,''/help/toolbox/simulink/help.jar!/slref/' lower(get_param(gcbh,'Blocktype')) '.html''], ''-helpbrowser''),end'])
      mask Display: plot([-0.05, 1.05, NaN, -0.05, 1.05],[.01, .01, NaN, .99, .99])
  mbtdisp1Enable_6 : Subsystem  Tag=et_enhanced_observability
      mask Type: MBT_DISP_BLOCK
      mask Display: text(0.1, 0.5, 'MBT_DISP')
  Out1 : Outport  InitialOutput=[0]
  wires:
  In1/1 -> Gain/1
  Gain/1 -> Out1/1
  Enable/1 -> mbtdisp1Enable_6/1(In)
  mbt_trigger_obs_1/1 -> mbt_trigger_obs_2/1
  mbt_trigger_obs_2/1 -> mbt_trigger_obs_1/1

== system ActionPort_obs/Subsystem/Subsystem/Subsystem/SubEnablePort/SubEnableVirtVect ==
  In1 : Inport
  Enable : EnablePort  ShowOutputPort=on
  Gain : Gain  mask(TL_Gain){data={'date',736495.67757076386}}
      settings: CopyFcn=if exist('tl_reset_reviewflag','file')==2,tl_reset_reviewflag(gcbh);end  DeleteFcn=if exist('delete_tlblock','file')==2,delete_tlblock(gcbh);end  NameChangeFcn=if exist('rename_tlblock','file')==2,rename_tlblock(gcbh);end  OpenFcn=if exist('tl_open_blockdlg','file')==2,tl_open_blockdlg(gcbh);else,open_system(gcbh,'parameter');end
      mask Help: eval(['if exist(''tl_online_help'',''file'') == 2, tl_online_help(''Topic'',''TL_Gain''),else, web([''jar:file:///'',matlabroot,''/help/toolbox/simulink/help.jar!/slref/' lower(get_param(gcbh,'Blocktype')) '.html''], ''-helpbrowser''),end'])
      mask Display: plot([0, .9, 0],[.05, .5, .95])
  mbt_trigger_obs_1 : Logic  Tag=mbt_add_trigger_obs  Operator=NOT  Inputs=1  AllPortsSameDT=off  OutDataTypeStr=boolean  mask(TL_LogicalOperator){data={'output',{'class','MBT_DISP'},'date',737456.3899889699}}
      settings: DeleteFcn=if exist('delete_tlblock','file')==2,delete_tlblock(gcbh);end  NameChangeFcn=if exist('rename_tlblock','file')==2,rename_tlblock(gcbh);end  OpenFcn=if exist('tl_open_blockdlg','file')==2,tl_open_blockdlg(gcbh);else,open_system(gcbh,'parameter');end
      mask Help: eval(['if exist(''tl_online_help'',''file'') == 2, tl_online_help(''Topic'',''TL_LogicalOperator''),else, web([''jar:file:///'',matlabroot,''/help/toolbox/simulink/help.jar!/slref/' lower(get_param(gcbh,'Blocktype')) '.html''], ''-helpbrowser''),end'])
      mask Display: plot([-0.05, 1.05, NaN, -0.05, 1.05],[.01, .01, NaN, .99, .99])
  mbt_trigger_obs_2 : UnitDelay  Tag=mbt_add_trigger_obs  SampleTime=-1  mask(TL_UnitDelay){data={'output',{'type','Bool'},'state',{'type','Bool'},'date',737456.3899895486}}
      settings: CopyFcn=if exist('tl_reset_reviewflag') == 2, tl_reset_reviewflag(gcbh); end  DeleteFcn=if exist('delete_tlblock','file')==2,delete_tlblock(gcbh);end  NameChangeFcn=if exist('rename_tlblock','file')==2,rename_tlblock(gcbh);end  OpenFcn=if exist('tl_open_blockdlg','file')==2,tl_open_blockdlg(gcbh);else,open_system(gcbh,'parameter');end
      mask Help: eval(['if exist(''tl_online_help'',''file'') == 2, tl_online_help(''Topic'',''TL_UnitDelay''),else, web([''jar:file:///'',matlabroot,''/help/toolbox/simulink/help.jar!/slref/' lower(get_param(gcbh,'Blocktype')) '.html''], ''-helpbrowser''),end'])
      mask Display: plot([-0.05, 1.05, NaN, -0.05, 1.05],[.01, .01, NaN, .99, .99])
  mbtdisp1Enable_2 : Subsystem  Tag=et_enhanced_observability
      mask Type: MBT_DISP_BLOCK
      mask Display: text(0.1, 0.5, 'MBT_DISP')
  Out1 : Outport  InitialOutput=[0]
  wires:
  In1/1 -> Gain/1
  Gain/1 -> Out1/1
  Enable/1 -> mbtdisp1Enable_2/1(In)
  mbt_trigger_obs_1/1 -> mbt_trigger_obs_2/1
  mbt_trigger_obs_2/1 -> mbt_trigger_obs_1/1
